simulink model "PolePlacement_with_noise_control"  (R2023a)
settings: Solver=ode4  StartTime=0.0  StopTime=10  FixedStep=0.001  RelTol=1e-3
InitFcn:
  | Init_control;
undefined symbols (not defined in the file): kpp, P, R, Ts
libraries: simulink x4
settings Model: Creator=wsh  LastModifiedBy=matte
settings SolverCC: AlgebraicLoopSolver=TrustRegion
settings DataIOCC: ReturnWorkspaceOutputs=off
settings DebuggingCC: UnconnectedInputMsg=warning  UnconnectedOutputMsg=warning  UnconnectedLineMsg=warning  BusObjectLabelMismatch=error  ArithmeticOperatorsInVariantConditions=warning
settings ModelReferenceCC: EnableRefExpFcnMdlSchedulingChecks=on
settings SFSimCC: SimUseLocalCustomCode=off  CustomCodeUndefinedFunction=UseInterfaceOnly
settings RTWCC: RTWUseLocalCustomCode=off
settings CodeAppCC: StateflowObjectComments=on

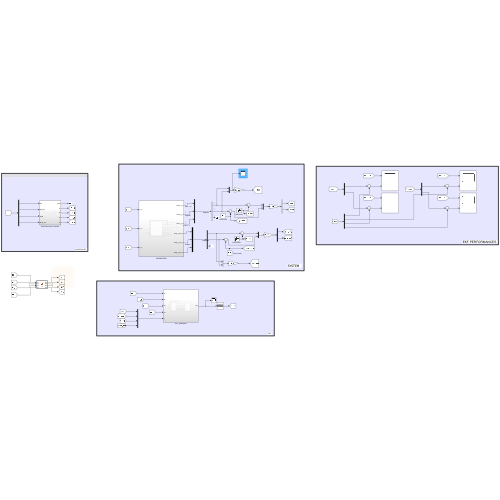
[thumbnail: Simulink's stored preview of the top-level diagram]
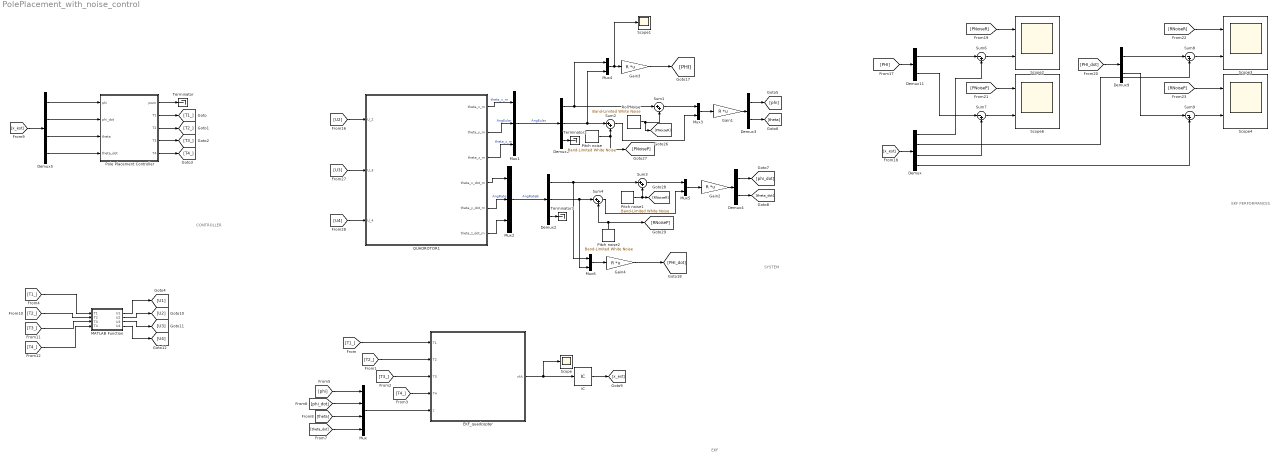
== system PolePlacement_with_noise_control ==
  note: CONTROLLER
  note: EKF PERFORMANCES
  note: EKF
  note: SYSTEM
  Demux : Demux
  Demux1 : Demux  Outputs=3
  Demux{3..4,9,11} (4 alike) : Demux  Outputs=2
  Demux2 : Demux  Outputs=3
  Demux5 : Demux
  EKF_quadcopter : Subsystem
  Gain{1..4} (4 alike) : Gain  Gain=R  Multiplication=Matrix(K*u) (u vector)
  IC : InitialCondition  Value=[0;0;0;0]
  MATLAB Function : MATLAB Function  TreatAsAtomicUnit=on
  Mux : Mux
  Mux1 : Mux  Inputs=3
  Mux2 : Mux  Inputs=3
  Mux{3..6} (4 alike) : Mux  Inputs=2
  Pitch noise : simulink/Sources/Band-Limited White Noise  Cov=[1.809123162388460e-08]  Ts=Ts  seed=[23341]
  Pitch noise1 : simulink/Sources/Band-Limited White Noise  Cov=[2.7827391e-06]  Ts=Ts  seed=[23341]
  Pitch noise2 : simulink/Sources/Band-Limited White Noise  Cov=[2.718240466492716e-06]  Ts=Ts  seed=[23341]
  Pole Placement Controller : Subsystem
  QUADROTOR1 : Subsystem
  Roll Noise : simulink/Sources/Band-Limited White Noise  Cov=[1.936548166270313e-08]  Ts=Ts  seed=[23341]
  Scope : Scope
  Scope1 : Scope
  Scope{2..4,6} (4 alike) : Scope  NumInputPorts=2
  Sum{1..4} (4 alike) : Sum  Inputs=|++
  Sum{6..9} (4 alike) : Sum  Inputs=|-+
  Terminator : Terminator
  Terminator2 : Terminator
  Terminator3 : Terminator
  wires:
  Pole Placement Controller/2(T1) -> [T1_]
  Pole Placement Controller/3(T2) -> [T2_]
  Pole Placement Controller/4(T3) -> [T3_]
  Pole Placement Controller/5(T4) -> [T4_]
  Demux5/1 -> Pole Placement Controller/1(phi)
  Demux5/2 -> Pole Placement Controller/2(phi_dot)
  Demux5/3 -> Pole Placement Controller/3(theta)
  Demux5/4 -> Pole Placement Controller/4(theta_dot)
  Pole Placement Controller/1(pwm) -> Terminator/1
  [x_est] -> Demux5/1
  Demux/3 -> Sum7/2
  Sum9/1 -> Scope4/2
  Demux/2 -> Sum8/2
  [PHI] -> Demux11/1
  Demux11/1 -> Sum6/1
  [x_est] -> Demux/1
  Sum7/1 -> Scope6/2
  [RNoiseP] -> Scope4/1
  [PNoiseP] -> Scope6/1
  Sum8/1 -> Scope3/2
  Demux/1 -> Sum6/2
  Demux/4 -> Sum9/2
  Mux/1 -> EKF_quadcopter/5(z)
  [theta] -> Mux/3
  Sum6/1 -> Scope2/2
  [T4_] -> EKF_quadcopter/4(T4)
  [phi] -> Mux/1
  [T2_] -> EKF_quadcopter/2(T2)
  [T3_] -> EKF_quadcopter/3(T3)
  Demux9/2 -> Sum9/1
  Demux11/2 -> Sum7/1
  [phi_dot] -> Mux/2
  IC/1 -> [x_est]
  [RNoiseR] -> Scope3/1
  EKF_quadcopter/1(xkk) -> IC/1, Scope/1
  [T1_] -> EKF_quadcopter/1(T1)
  [PNoiseR] -> Scope2/1
  [theta_dot] -> Mux/4
  Demux9/1 -> Sum8/1
  [PHI_dot] -> Demux9/1
  QUADROTOR1/1(theta_x_m) -> Mux1/1  "theta_x_m"
  [U4] -> QUADROTOR1/3(U_4)
  QUADROTOR1/5(theta_y_dot_m) -> Mux2/2  "AngRate"
  [U2] -> QUADROTOR1/1(U_2)
  QUADROTOR1/4(theta_x_dot_m) -> Mux2/1
  QUADROTOR1/2(theta_y_m) -> Mux1/2  "AngEular"
  [U3] -> QUADROTOR1/2(U_3)
  QUADROTOR1/3(theta_z_m) -> Mux1/3  "theta_z_m"
  QUADROTOR1/6(theta_z_dot_m) -> Mux2/3
  Demux1/3 -> Terminator2/1
  Demux4/2 -> [theta_dot]
  Sum2/1 -> Mux3/2
  Demux4/1 -> [phi_dot]
  Sum4/1 -> Mux5/2
  Pitch noise/1 -> [PNoiseP], Sum2/2
  Gain4/1 -> [PHI_dot]
  Pitch noise2/1 -> [RNoiseP], Sum4/2
  Demux3/2 -> [theta]
  Demux3/1 -> [phi]
  Demux2/3 -> Terminator3/1
  Sum3/1 -> Mux5/1
  Demux2/2 -> Mux6/2, Sum4/1
  Roll Noise/1 -> [PNoiseR], Sum1/2
  Mux3/1 -> Gain1/1
  Sum1/1 -> Mux3/1
  Mux6/1 -> Gain4/1
  Gain1/1 -> Demux3/1
  Gain2/1 -> Demux4/1
  Mux5/1 -> Gain2/1
  Demux2/1 -> Mux6/1, Sum3/1
  Mux1/1 -> Demux1/1  "AngEular"
  Demux1/2 -> Mux4/2, Sum2/1
  Pitch noise1/1 -> [RNoiseR], Sum3/2
  Demux1/1 -> Mux4/1, Sum1/1
  Mux2/1 -> Demux2/1  "AngRateB"
  Mux4/1 -> Scope1/1, Gain3/1
  Gain3/1 -> [PHI]
  [T1_] -> MATLAB Function/1(T1)
  [T2_] -> MATLAB Function/2(T2)
  [T3_] -> MATLAB Function/3(T3)
  [T4_] -> MATLAB Function/4(T4)
  MATLAB Function/1(U1) -> [U1]
  MATLAB Function/2(U2) -> [U2]
  MATLAB Function/3(U3) -> [U3]
  MATLAB Function/4(U4) -> [U4]

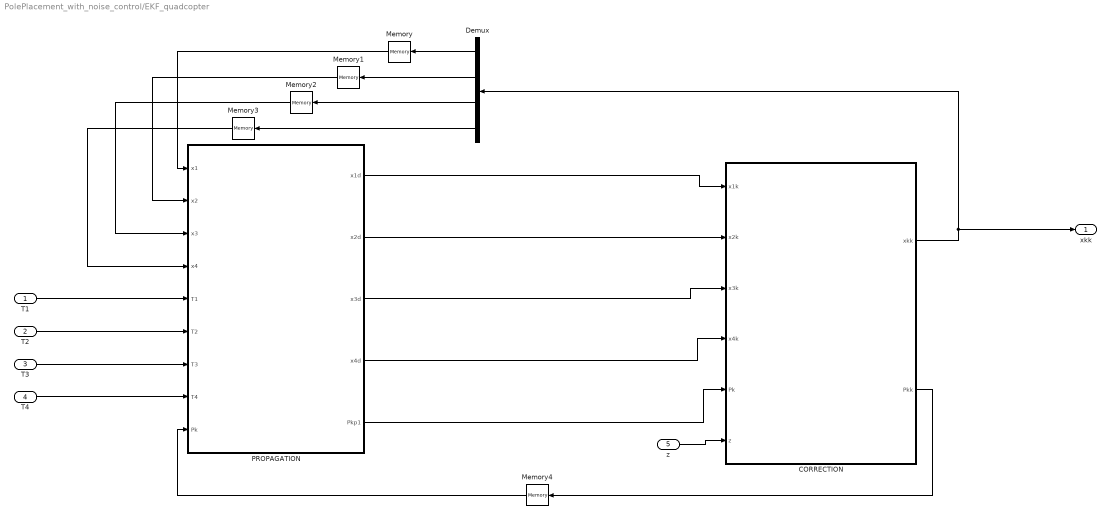
== system PolePlacement_with_noise_control/EKF_quadcopter ==
  T1 : Inport
  T2 : Inport  Port=2
  T3 : Inport  Port=3
  T4 : Inport  Port=4
  z : Inport  Port=5
  CORRECTION : MATLAB Function  TreatAsAtomicUnit=on
  Demux : Demux
  Memory{,1..3} (4 alike) : Memory
  Memory4 : Memory  InitialCondition=P
  PROPAGATION : MATLAB Function  TreatAsAtomicUnit=on
  xkk : Outport
  wires:
  PROPAGATION/1(x1d) -> CORRECTION/1(x1k)
  PROPAGATION/2(x2d) -> CORRECTION/2(x2k)
  PROPAGATION/3(x3d) -> CORRECTION/3(x3k)
  PROPAGATION/4(x4d) -> CORRECTION/4(x4k)
  Memory4/1 -> PROPAGATION/9(Pk)
  T1/1 -> PROPAGATION/5(T1)
  T2/1 -> PROPAGATION/6(T2)
  T3/1 -> PROPAGATION/7(T3)
  T4/1 -> PROPAGATION/8(T4)
  PROPAGATION/5(Pkp1) -> CORRECTION/5(Pk)
  CORRECTION/2(Pkk) -> Memory4/1
  z/1 -> CORRECTION/6(z)
  Demux/1 -> Memory/1
  Demux/2 -> Memory1/1
  Demux/3 -> Memory2/1
  Demux/4 -> Memory3/1
  CORRECTION/1(xkk) -> Demux/1, xkk/1
  Memory/1 -> PROPAGATION/1(x1)
  Memory1/1 -> PROPAGATION/2(x2)
  Memory2/1 -> PROPAGATION/3(x3)
  Memory3/1 -> PROPAGATION/4(x4)

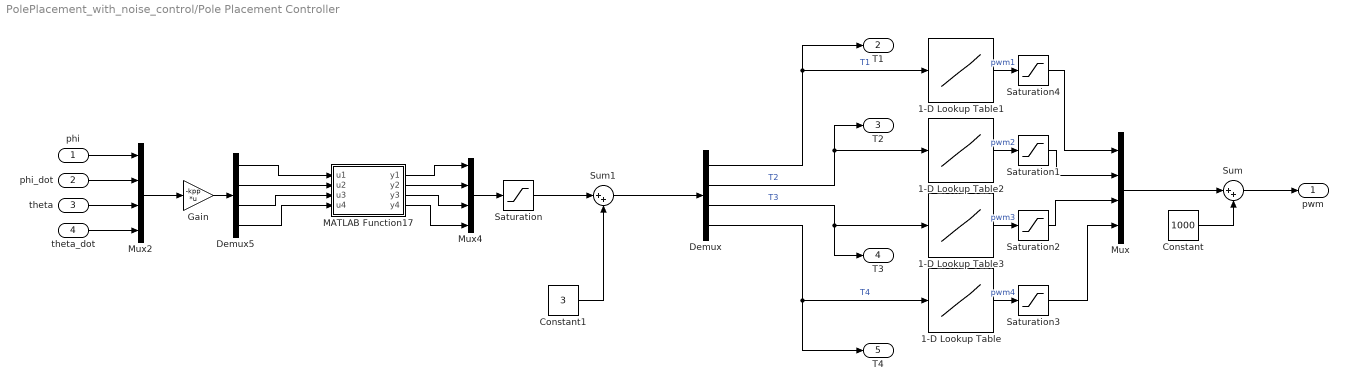
== system PolePlacement_with_noise_control/Pole Placement Controller ==
  phi : Inport
  phi_dot : Inport  Port=2
  theta : Inport  Port=3
  theta_dot : Inport  Port=4
  1-D Lookup Table : Lookup_n-D  NumberOfTableDimensions=1  BreakpointsForDimension1=[0;0.06477642396;0.16;0.63;2.44;4.43;6.92;8.77;10.52;11.63;12.03;12.09;12.091;12.092;12.093;12.094;12.095;12.096;12.097;12.098;12.099]  Table=[0;50;100;150;200;250;300;350;400;450;500;550;600;650;700;750;800;850;900;950;1000]  InternalRulePriority=Speed  RndMeth=Simplest
  1-D Lookup Table1 : Lookup_n-D  NumberOfTableDimensions=1  BreakpointsForDimension1=[0;0.02;0.06;0.29;0.73;1.07;1.88;2.91;4;5.06;6.71;7.86;9.41;10.86;11.45;11.82;12.07;12.31;12.52;12.74;12.75]  Table=[0;50;100;150;200;250;300;350;400;450;500;550;600;650;700;750;800;850;900;950;1000]  InternalRulePriority=Speed  RndMeth=Simplest
  1-D Lookup Table2 : Lookup_n-D  NumberOfTableDimensions=1  BreakpointsForDimension1=[0;0.05;0.39;1.67;3.19;5.57;8.07;10.01;10.71;11.06;11.42;11.53;11.55;11.551;11.552;11.553;11.554;11.555;11.556;11.557;11.558]  Table=[0;50;100;150;200;250;300;350;400;450;500;550;600;650;700;750;800;850;900;950;1000]  InternalRulePriority=Speed  RndMeth=Simplest
  1-D Lookup Table3 : Lookup_n-D  NumberOfTableDimensions=1  BreakpointsForDimension1=[0;0.06;0.23;0.89;2.47;3.9;5.86;7.81;9.42;10.12;10.6;11.01;11.34;11.39;11.391;11.392;11.393;11.394;11.395;11.396;11.397]  Table=[0;50;100;150;200;250;300;350;400;450;500;550;600;650;700;750;800;850;900;950;1000]  InternalRulePriority=Speed  RndMeth=Simplest
  Constant : Constant  Value=1000
  Constant1 : Constant  Value=3
  Demux : Demux
  Demux5 : Demux
  Gain : Gain  Gain=-kpp  Multiplication=Matrix(K*u) (u vector)
  MATLAB Function17 : MATLAB Function  TreatAsAtomicUnit=on
  Mux : Mux
  Mux2 : Mux
  Mux4 : Mux
  Saturation : Saturate  UpperLimit=10  LowerLimit=0
  Saturation{1..4} (4 alike) : Saturate  UpperLimit=1000  LowerLimit=0
  Sum : Sum  Inputs=|++
  Sum1 : Sum  Inputs=|++
  pwm : Outport
  T1 : Outport  Port=2
  T2 : Outport  Port=3
  T3 : Outport  Port=4
  T4 : Outport  Port=5
  wires:
  Mux4/1 -> Saturation/1
  Mux2/1 -> Gain/1
  theta/1 -> Mux2/3
  1-D Lookup Table1/1 -> Saturation4/1  "pwm1"
  Saturation/1 -> Sum1/1
  Constant1/1 -> Sum1/2
  phi/1 -> Mux2/1
  1-D Lookup Table/1 -> Saturation3/1  "pwm4"
  Saturation4/1 -> Mux/1
  Demux5/2 -> MATLAB Function17/2(u2)
  Demux/1 -> T1/1, 1-D Lookup Table1/1  "T1"
  Gain/1 -> Demux5/1
  Saturation2/1 -> Mux/3
  Demux/4 -> T4/1, 1-D Lookup Table/1  "T4"
  Demux/3 -> T3/1, 1-D Lookup Table3/1  "T3"
  Demux5/4 -> MATLAB Function17/4(u4)
  Saturation1/1 -> Mux/2
  1-D Lookup Table3/1 -> Saturation2/1  "pwm3"
  Demux/2 -> 1-D Lookup Table2/1, T2/1  "T2"
  Sum1/1 -> Demux/1
  1-D Lookup Table2/1 -> Saturation1/1  "pwm2"
  MATLAB Function17/2(y2) -> Mux4/2
  Saturation3/1 -> Mux/4
  Demux5/3 -> MATLAB Function17/3(u3)
  MATLAB Function17/3(y3) -> Mux4/3
  MATLAB Function17/1(y1) -> Mux4/1
  MATLAB Function17/4(y4) -> Mux4/4
  Demux5/1 -> MATLAB Function17/1(u1)
  phi_dot/1 -> Mux2/2
  theta_dot/1 -> Mux2/4
  Sum/1 -> pwm/1
  Mux/1 -> Sum/1
  Constant/1 -> Sum/2

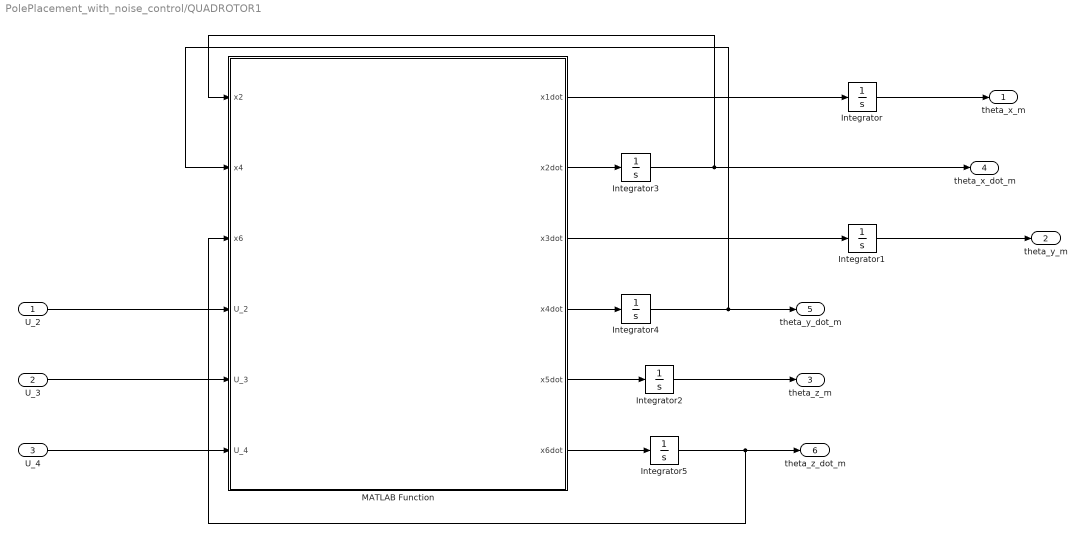
== system PolePlacement_with_noise_control/QUADROTOR1 ==
  U_2 : Inport
  U_3 : Inport  Port=2
  U_4 : Inport  Port=3
  Integrator : Integrator  InitialCondition=0.4
  Integrator1 : Integrator  InitialCondition=0.3
  Integrator2 : Integrator  InitialCondition=-0.2
  Integrator3 : Integrator
  Integrator4 : Integrator
  Integrator5 : Integrator
  MATLAB Function : MATLAB Function  TreatAsAtomicUnit=on
  theta_x_m : Outport
  theta_y_m : Outport  Port=2
  theta_z_m : Outport  Port=3
  theta_x_dot_m : Outport  Port=4
  theta_y_dot_m : Outport  Port=5
  theta_z_dot_m : Outport  Port=6
  wires:
  U_2/1 -> MATLAB Function/4(U_2)
  U_3/1 -> MATLAB Function/5(U_3)
  U_4/1 -> MATLAB Function/6(U_4)
  MATLAB Function/3(x3dot) -> Integrator1/1
  MATLAB Function/5(x5dot) -> Integrator2/1
  MATLAB Function/2(x2dot) -> Integrator3/1
  MATLAB Function/4(x4dot) -> Integrator4/1
  MATLAB Function/6(x6dot) -> Integrator5/1
  Integrator/1 -> theta_x_m/1
  MATLAB Function/1(x1dot) -> Integrator/1
  Integrator1/1 -> theta_y_m/1
  Integrator2/1 -> theta_z_m/1
  Integrator5/1 -> theta_z_dot_m/1, MATLAB Function/3(x6)
  Integrator4/1 -> MATLAB Function/2(x4), theta_y_dot_m/1
  Integrator3/1 -> MATLAB Function/1(x2), theta_x_dot_m/1

== matlab function PolePlacement_with_noise_control/EKF_quadcopter/CORRECTION ==
  data: x1k input; xkk output; Pkk output; x2k input; x3k input; x4k input; Pk input; z input
function [xkk,Pkk] = fcn(x1k,x2k,x3k,x4k,Pk,z)

R = [1.936548166270313e-08 0 0 0;
     0 2.7827391e-06 0 0;
     0 0 1.809123162388460e-08 0;
     0 0 0 2.718240466492716e-06];

H = [1 0 0 0;
     0 1 0 0;
     0 0 1 0;
     0 0 0 1];

xk = [x1k;x2k;x3k;x4k];

y = z - H * xk;

K = Pk*(H')/(H*Pk*(H') + R);

xkk = xk + K * y;
Pkk = (eye(4)-K * H) * Pk;

== matlab function PolePlacement_with_noise_control/EKF_quadcopter/PROPAGATION ==
  data: x1 input; x1d output; x2 input; x3 input; x4 input; T1 input; T2 input; T3 input; T4 input; x2d output; x3d output; x4d output; Pk input; Pkp1 output
function [x1d,x2d,x3d,x4d,Pkp1] = fcn(x1,x2,x3,x4,T1,T2,T3,T4,Pk)

m = 1.07;
L = 0.25;
d = 0.055;
J = 0.055;
g = 9.81;
Ts = 0.002;

Q = [1e-7 0 0 0;
     0 1e-4 0 0;
     0 0 1e-10 0;
     0 0 0 1e-7];

F11 = 0;
F12 = 1;
F13 = 0;
F14 = 0;

F21 = m*g*d/J*cos(x1)+T2*(-L*sin(x1)-d*cos(x1))/J-T1*(-L*sin(x1)+d*cos(x1))/J;
F22 = 0;
F23 = 0;
F24 = 0;

F31 = 0;
F32 = 0;
F33 = 0;
F34 = 1;


F41 = 0;
F42 = 0;
F43 = m*g*d*cos(x3)/J+T4*(-L*sin(x3)-d*cos(x3))/J-T3*(-L*sin(x3)+d*cos(x3))/J;
F44 = 0;

F = [F11 F12 F13 F14;
     F21 F22 F23 F24;
     F31 F32 F33 F34;
     F41 F42 F43 F44];

PHI = expm(F * Ts);

x1d_dot = x2;
x2d_dot = m*g*d*sin(x1)/J + T2*(L*cos(x1)-d*sin(x1))/J - T1*(L*cos(x1) + ...
    d*sin(x1))/J;
x3d_dot = x4;
x4d_dot = m*g*d*sin(x3)/J + T4*(L*cos(x3)-d*sin(x3))/J - T3*(L*cos(x3) + ...
    d*sin(x3))/J;

x1d = x1 + x1d_dot*Ts;
x2d = x2 + x2d_dot*Ts;
x3d = x3 + x3d_dot*Ts;
x4d = x4 + x4d_dot*Ts;

Pkp1 = PHI * Pk * (PHI') + Q;

== matlab function PolePlacement_with_noise_control/MATLAB Function ==
  data: T1 input; U1 output; T2 input; T3 input; T4 input; U2 output; U3 output; U4 output
function [U1,U2,U3,U4] = fcn(T1,T2,T3,T4)


L = 0.2121;
kd= 1.779e-07;
kt = 1.105e-05;

U = [1             1           1            1;
    -L*sqrt(2)/2  L*sqrt(2)/2  L*sqrt(2)/2  -L*sqrt(2)/2;
    L*sqrt(2)/2  -L*sqrt(2)/2  L*sqrt(2)/2  -L*sqrt(2)/2;
    kd/kt            kd/kt       -kd/kt       -kd/kt    ] *[T1;T2;T3;T4];

U1 = U(1);
U2 = U(2);
U3 = U(3);
U4 = U(4);

== matlab function PolePlacement_with_noise_control/QUADROTOR1/MATLAB Function ==
  data: x2 input; x4 input; x6 input; x1dot output; U_2 input; U_3 input; U_4 input; x2dot output; x3dot output; x4dot output; x5dot output; x6dot output; quadParams parameter
function [x1dot,x2dot,x3dot,x4dot,x5dot,x6dot]= fcn(x2,x4,x6,U_2,U_3,U_4,quadParams)

a1=(quadParams.Jy-quadParams.Jz)/quadParams.Jx;
a2=-quadParams.Jr/quadParams.Jx;
a3=(quadParams.Jz-quadParams.Jx)/quadParams.Jy;
a4=quadParams.Jr/quadParams.Jy;
a5=(quadParams.Jx-quadParams.Jy)/quadParams.Jz;
b1=quadParams.L/quadParams.Jx;
b2=quadParams.L/quadParams.Jy;
b3=quadParams.L/quadParams.Jz;


x1dot=x2;

x2dot=x4*x6*a1 + b1*U_2;

x3dot=x4;

x4dot=x2*x6*a3+b2*U_3;

x5dot=x6;

x6dot=x4*x2*a5+b3*U_4;

== matlab function PolePlacement_with_noise_control/Pole Placement Controller/MATLAB Function17 ==
  data: u1 input; y1 output; u2 input; u3 input; u4 input; y2 output; y3 output; y4 output
function [y1,y2,y3,y4] = fcn(u1,u2,u3,u4)

if u1 < 0
    u2 = u2 + abs(u1);
    u1 = u1+abs(u1);
end
if u2 < 0
    u2 = u2 + abs(u2);
    u1 = u1 + abs(u2);
end
if u3 < 0
    u3 = u3 + abs(u3);
    u4 = u4 + abs(u3);
end    
if u4 < 0
    u4 = u4 + abs(u4);
    u3 = u3 + abs(u4);
end
 y1 = u1;
 y2 = u2;
 y3 = u3;
 y4 = u4;
